simulink model "plant_setup"  (R2022b)
settings: Solver=VariableStepAuto  StartTime=0.0  StopTime=10  RelTol=1e-3
model workspace (MAT data in the model file):
  T_max = Simulink.Parameter
  T_max.Value = 10
  T_max.Description = 'maximum allowable torque command'
  T_max.DataType = 'auto'
  T_max.DocUnits = 'N*m'
  T_max.Complexity = 'real'
  T_max.Dimensions = [1 1]
  bw = Simulink.Parameter
  bw.Value = 0.24
  bw.Description = 'Distance between the two drive wheels'
  bw.DataType = 'auto'
  bw.DocUnits = 'm'
  bw.Complexity = 'real'
  bw.Dimensions = [1 1]
  k_D = Simulink.Parameter
  k_D.Value = 1
  k_D.DataType = 'auto'
  k_D.Complexity = 'real'
  k_D.Dimensions = [1 1]
  k_P = Simulink.Parameter
  k_P.Value = Simulink.data.Expression
  k_P.Value.ExpressionString = "20*k_D"
  k_P.DataType = 'auto'
  k_P.Complexity = 'real'
  k_P.Dimensions = -1
  r_turn = Simulink.Parameter
  r_turn.Value = 0.2
  r_turn.Description = 'Minimum turn radius of the car'
  r_turn.DataType = 'auto'
  r_turn.Min = 0
  r_turn.DocUnits = 'm'
  r_turn.Complexity = 'real'
  r_turn.Dimensions = [1 1]
  r_wheel = Simulink.Parameter
  r_wheel.Value = 0.11
  r_wheel.Description = 'Wheel radius'
  r_wheel.DataType = 'auto'
  r_wheel.DocUnits = 'm'
  r_wheel.Complexity = 'real'
  r_wheel.Dimensions = [1 1]
  v_base = Simulink.Parameter
  v_base.Value = 0.5
  v_base.Description = 'base wheel speed (m/s) used for turns
    | v_base = w_turn_max 8 bw/2'
  v_base.DataType = 'auto'
  v_base.DocUnits = 'm/s'
  v_base.Complexity = 'real'
  v_base.Dimensions = [1 1]
  v_max = Simulink.Parameter
  v_max.Value = 1
  v_max.Description = 'max car speed in m/s'
  v_max.DataType = 'auto'
  v_max.DocUnits = 'm/s'
  v_max.Complexity = 'real'
  v_max.Dimensions = [1 1]
  w_max = Simulink.Parameter
  w_max.Value = Simulink.data.Expression
  w_max.Value.ExpressionString = "9.0909*v_max"
  w_max.Description = 'max wheel speed in rad/s
    | w_max = v_max/r_wheel'
  w_max.DataType = 'auto'
  w_max.DocUnits = 'rad/s'
  w_max.Complexity = 'real'
  w_max.Dimensions = -1
  w_turn_max = Simulink.Parameter
  w_turn_max.Value = 4
  w_turn_max.Description = 'max turning speed of car in rad/s
    | w_turn_max = w_max * r_wheel/bw'
  w_turn_max.DataType = 'auto'
  w_turn_max.DocUnits = 'rad/s'
  w_turn_max.Complexity = 'real'
  w_turn_max.Dimensions = [1 1]
undefined symbols (not defined in the file or in its folder): duration, effort, index, joint_name, left_wheel_hinge, model_name, pioneer2dx, right_wheel_hinge
libraries: robotgazebolib x21, robotcorelib x1, simulink x1
settings Model: Creator=22546723@sun.ac.za  LastModifiedBy=22546723@sun.ac.za

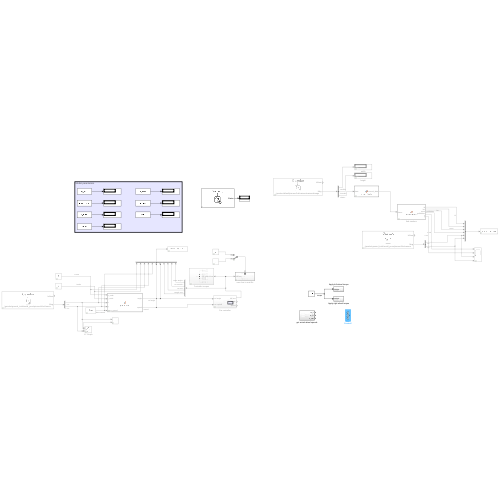
[thumbnail: Simulink's stored preview of the top-level diagram]
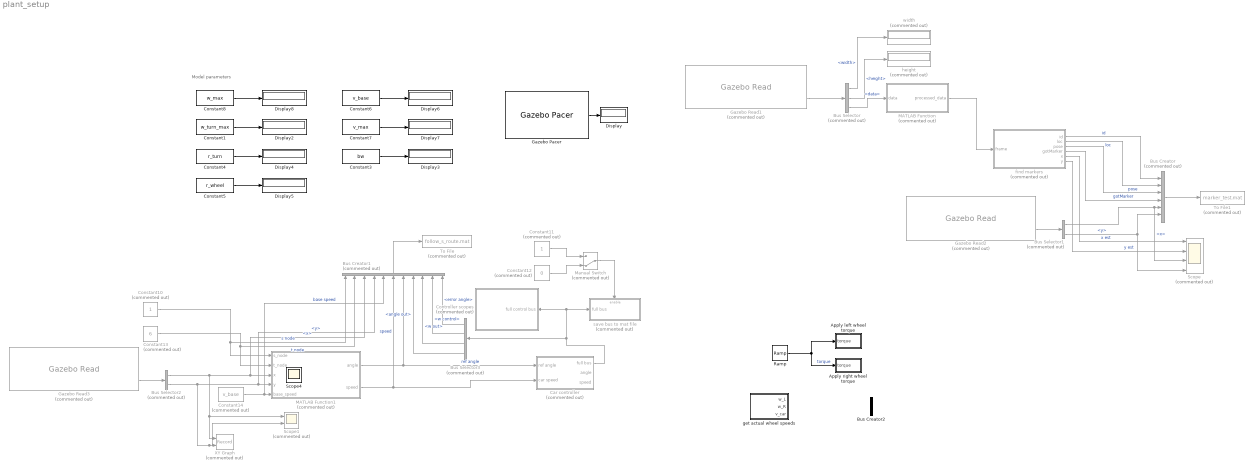
== system plant_setup ==
  note: Model parameters
  Apply left wheel torque : Subsystem
  Apply right wheel torque : Subsystem
  Bus Creator : BusCreator  Commented=on  Inputs=6
  Bus Creator1 : BusCreator  Commented=on  Inputs=11
  Bus Creator2 : BusCreator  Inputs=2
  Bus Selector : BusSelector  Commented=on  OutputSignals=width,height,data
  Bus Selector1 : BusSelector  Commented=on  OutputSignals=position.x,position.y
  Bus Selector2 : BusSelector  Commented=on  OutputSignals=position.x,position.y
  Bus Selector3 : BusSelector  Commented=on  OutputSignals=error angle,w control,w out,angle out
  Car controller : Subsystem  Commented=on
  Constant1 : Constant  Value=w_turn_max
  Constant10 : Constant  Commented=on
  Constant11 : Constant  Commented=on
  Constant12 : Constant  Commented=on  Value=0
  Constant13 : Constant  Commented=on  Value=6
  Constant14 : Constant  Commented=on  Value=v_base
  Constant3 : Constant  Value=bw
  Constant4 : Constant  Value=r_turn
  Constant5 : Constant  Value=r_wheel
  Constant6 : Constant  Value=v_base
  Constant7 : Constant  Value=v_max
  Constant8 : Constant  Value=w_max
  Controller scopes : Subsystem  Commented=on
      settings: PortSchema="{\"entries\":[{\"content\":{\"sides\":[{\"content\":{\"connectorIds\":[]},\"type\":\"ConnectorPlacement.EquallySpacedRectSide\",\"uuid\":\"333996ec-a739-4064-b7cd-e5a785ad06b0\"},{\"content\":{\"connectorIds\":[\"In1\"],\"side\":\"RIGHT\"},\"type\":\"ConnectorPlacement.EquallySpacedRectSide\",\"uuid\":\"5c2099fd-2913-4b55-a92e-2fa47d7778a9\"},{\"content\":{\"connectorIds\":[],\"side\":\"TOP\"},\"type\":\"ConnectorPlacement.EquallySpacedRectSide\",\"uuid\":\"27960070-26ba-4880-ac4a-dbd824c43cf7\"}]},\"type\":\"ConnectorPlacement.EquallySpacedConnector\",\"uuid\":\"80cd80e5-3dd6-4d73-8038-72b1cdb99f2f\"}],\"packageUris\":[\"http://schema.mathworks.com/mf0/Connector/R2020b\"],\"version\":\"1.0\"}"
  Display{,2..8} (8 alike) : Display
  Gazebo Pacer : robotgazebolib/Gazebo Pacer  ResetBehavior=Reset Gazebo simulation time  SampleTime=0.001
  Gazebo Read1 : robotgazebolib/Gazebo Read  Commented=on  topicSource=From Gazebo  topic=/gazebo/default/pioneer2dx/camera/camera/image  messageType=gazebo_msgs/Image  sampleTime=0.001  fixedAxisBusStatus=off  jointAxisCount=2
  Gazebo Read2 : robotgazebolib/Gazebo Read  Commented=on  topicSource=From Gazebo  topic=/gazebo/ground_truth/world_pose/pioneer2dx/camera  messageType=gazebo_msgs/Pose  sampleTime=0.001  fixedAxisBusStatus=off  jointAxisCount=2
  Gazebo Read3 : robotgazebolib/Gazebo Read  Commented=on  topicSource=From Gazebo  topic=/gazebo/ground_truth/world_pose/pioneer2dx/chassis  messageType=gazebo_msgs/Pose  sampleTime=0.001  fixedAxisBusStatus=off  jointAxisCount=2
  MATLAB Function : MATLAB Function  Commented=on  TreatAsAtomicUnit=on
  MATLAB Function1 : MATLAB Function  Commented=on  TreatAsAtomicUnit=on
  Manual Switch : ManualSwitch  Commented=on  CurrentSetting=0
  Ramp : simulink/Sources/Ramp  slope=1  start=0  InitialOutput=0
  Scope : Scope  Commented=on  NumInputPorts=4
  Scope1 : Scope  Commented=on  NumInputPorts=2
  To File : ToFile  Commented=on  Filename=follow_s_route.mat  MatrixName=data  SaveFormat=Timeseries
  To File1 : ToFile  Commented=on  Filename=marker_test.mat  MatrixName=data  SaveFormat=Timeseries
  XY Graph : Record  Commented=on  FileSettingsInternal="{\"entries\":[{\"content\":{\"excelSettings\":{\"content\":{},\"type\":\"Streamout.ExcelSettings\"}},\"type\":\"Streamout.FileSettingStorage\",\"uuid\":\"0a0b0592-9645-4dd3-85ce-6b555624b077\"}],\"packageUris\":[\"http://schema.mathworks.com/mf0/streamout_blocks/R2020a\"],\"version\":\"1.0\"}"  Layout=[1 1]  SignalsInternal="{\"entries\":[{\"content\":{\"signals\":[{\"content\":{\"blockPath\":[\"plant_setup/XY Graph\"],\"channel\":[],\"dimensions\":[1],\"domain\":\"plant_setup/XY Graph\",\"lineColor\":\"#a2142f\",\"plots\":[1],\"port\":1,\"sid\":[],\"signalID\":8,\"signalName\":\"<x>\"},\"type\":\"RecordBlkView.Signal\",\"uuid\":\"999196a1-9528-4da5-9067-52614dff8acd\"},{\"content\":{\"blockPath\":[\"plant_setup/XY Graph\"],\"channel\":[],\"dimensions\":[1],\"domain\":\"plant_setup/XY Graph\",\"lineColor\":\"#139fff\",\"plots\":[1],\"port\":2,\"sid\":[],\"signalID\":11,\"signalName\":\"<y>\"},\"type\":\"RecordBlkView.Signal\",\"uuid\":\"a6f77fcf-062b-42f5-9d76-fad9be37ea72\"}]},\"type\":\"RecordBlkView.InputSignals\",\"uuid\":\"03c2072b-3f6b-465e-b664-df38b8c2c7b2\"}],\"packageUris\":[\"http://schema.mathworks.com/mf0/streamout_blocks/R2020a\"],\"version\":\"1.0\"}"  VisualizationBindings="{\"xyplotplugin\":{\"info\":[{\"series\":[{\"bindingParametersList\":[{\"parameter\":\"X-Axis\",\"signalID\":8,\"signalName\":\"<x>\"},{\"parameter\":\"Y-Axis\",\"signalID\":11,\"signalName\":\"<y>\"}],\"seriesID\":29853}],\"subplotID\":1}]}}"  CompatibilityTag=XY
  find markers : MATLAB Function  Commented=on  TreatAsAtomicUnit=on
  get actual wheel speeds : Subsystem
  height : Display  Commented=on
  save bus to mat file : Subsystem  Commented=on  TreatAsAtomicUnit=on
  width : Display  Commented=on
  Scope4 : Scope
  wires:
  Gazebo Pacer/1 -> Display/1
  Constant1/1 -> Display2/1
  Constant3/1 -> Display3/1
  Constant4/1 -> Display4/1
  Constant5/1 -> Display5/1
  Constant6/1 -> Display6/1
  Constant7/1 -> Display7/1
  Constant8/1 -> Display8/1
  Car controller/1(full bus) -> Bus Selector3/1, save bus to mat file/1(full bus), Controller scopes/1(full control bus)
  Gazebo Read1/2 -> Bus Selector/1
  Bus Selector/3 -> MATLAB Function/1(data)  "<data>"
  Gazebo Read2/2 -> Bus Selector1/1
  find markers/3(pose) -> Bus Creator/3  "pose"
  find markers/4(gotMarker) -> Bus Creator/4  "gotMarker"
  Bus Selector1/1 -> Scope/3, Bus Creator/5  "<x>"
  Bus Selector1/2 -> Scope/4, Bus Creator/6  "<y>"
  MATLAB Function/1(processed_data) -> find markers/1(frame)
  Bus Creator/1 -> To File1/1
  find markers/2(loc) -> Bus Creator/2  "loc"
  find markers/1(id) -> Bus Creator/1  "id"
  Constant11/1 -> Manual Switch/1
  Constant12/1 -> Manual Switch/2
  Manual Switch/1 -> save bus to mat file/Enable
  Bus Selector/1 -> width/1  "<width>"
  Bus Selector/2 -> height/1  "<height>"
  find markers/5(x) -> Scope/1  "x est"
  find markers/6(y) -> Scope/2  "y est"
  Constant10/1 -> MATLAB Function1/1(s_node), Bus Creator1/1  "s node"
  Constant13/1 -> MATLAB Function1/2(t_node), Bus Creator1/2  "t node"
  MATLAB Function1/2(speed) -> Bus Creator1/6, Car controller/2(car speed)  "speed"
  Constant14/1 -> Bus Creator1/5, MATLAB Function1/5(base_speed)  "base speed"
  Gazebo Read3/2 -> Bus Selector2/1
  Bus Selector2/1 -> Scope1/1, XY Graph/1, MATLAB Function1/3(x), Bus Creator1/3  "<x>"
  Bus Selector2/2 -> Scope1/2, XY Graph/2, MATLAB Function1/4(y), Bus Creator1/4  "<y>"
  MATLAB Function1/1(angle) -> Bus Creator1/7, Car controller/1(ref angle)  "ref angle"
  Bus Selector3/1 -> Bus Creator1/11  "<error angle>"
  Bus Selector3/2 -> Bus Creator1/10  "<w control>"
  Bus Selector3/3 -> Bus Creator1/9  "<w out>"
  Bus Selector3/4 -> Bus Creator1/8  "<angle out>"
  Bus Creator1/1 -> To File/1
  Ramp/1 -> Apply right wheel torque/1(torque), Apply left wheel torque/1(torque)  "torque"

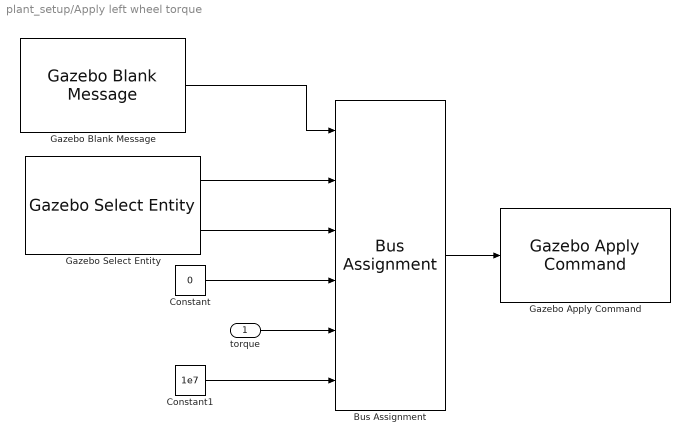
== system plant_setup/Apply left wheel torque ==
  torque : Inport  SampleTime=0.001
  Bus Assignment : BusAssignment  AssignedSignals=model_name,joint_name,index,effort,duration.nano_seconds
  Constant : Constant  Value=0  OutDataTypeStr=uint32  SampleTime=0.001
  Constant1 : Constant  Value=1e7  SampleTime=0.001
  Gazebo Apply Command : robotgazebolib/Gazebo Apply Command  cmdType=ApplyJointTorque  sampleTime=0.001
  Gazebo Blank Message : robotgazebolib/Gazebo Blank Message  msgType=ApplyJointTorque  sampleTime=0.001  busName='Gazebo_SL_Bus_gazebo_msgs_ApplyJointTorque'
  Gazebo Select Entity : robotgazebolib/Gazebo Select Entity  modelElemName=pioneer2dx/left_wheel_hinge  outputArraySize=128  OutputLabel=Joint  SelectType=Joint
  wires:
  Gazebo Select Entity/1 -> Bus Assignment/2
  Bus Assignment/1 -> Gazebo Apply Command/1
  Gazebo Blank Message/1 -> Bus Assignment/1
  Constant/1 -> Bus Assignment/4
  Gazebo Select Entity/2 -> Bus Assignment/3
  Constant1/1 -> Bus Assignment/6
  torque/1 -> Bus Assignment/5

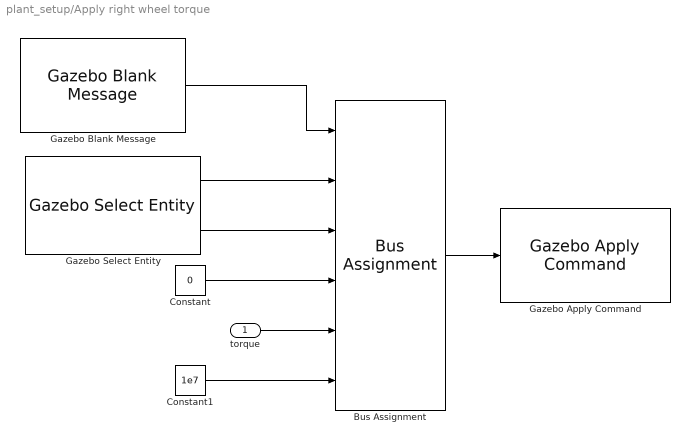
== system plant_setup/Apply right wheel torque ==
  torque : Inport  SampleTime=0.001
  Bus Assignment : BusAssignment  AssignedSignals=model_name,joint_name,index,effort,duration.nano_seconds
  Constant : Constant  Value=0  OutDataTypeStr=uint32  SampleTime=0.001
  Constant1 : Constant  Value=1e7  SampleTime=0.001
  Gazebo Apply Command : robotgazebolib/Gazebo Apply Command  cmdType=ApplyJointTorque  sampleTime=0.001
  Gazebo Blank Message : robotgazebolib/Gazebo Blank Message  msgType=ApplyJointTorque  sampleTime=0.001  busName='Gazebo_SL_Bus_gazebo_msgs_ApplyJointTorque'
  Gazebo Select Entity : robotgazebolib/Gazebo Select Entity  modelElemName=pioneer2dx/right_wheel_hinge  outputArraySize=128  OutputLabel=Joint  SelectType=Joint
  wires:
  Gazebo Select Entity/1 -> Bus Assignment/2
  Bus Assignment/1 -> Gazebo Apply Command/1
  Gazebo Blank Message/1 -> Bus Assignment/1
  Constant/1 -> Bus Assignment/4
  Gazebo Select Entity/2 -> Bus Assignment/3
  Constant1/1 -> Bus Assignment/6
  torque/1 -> Bus Assignment/5

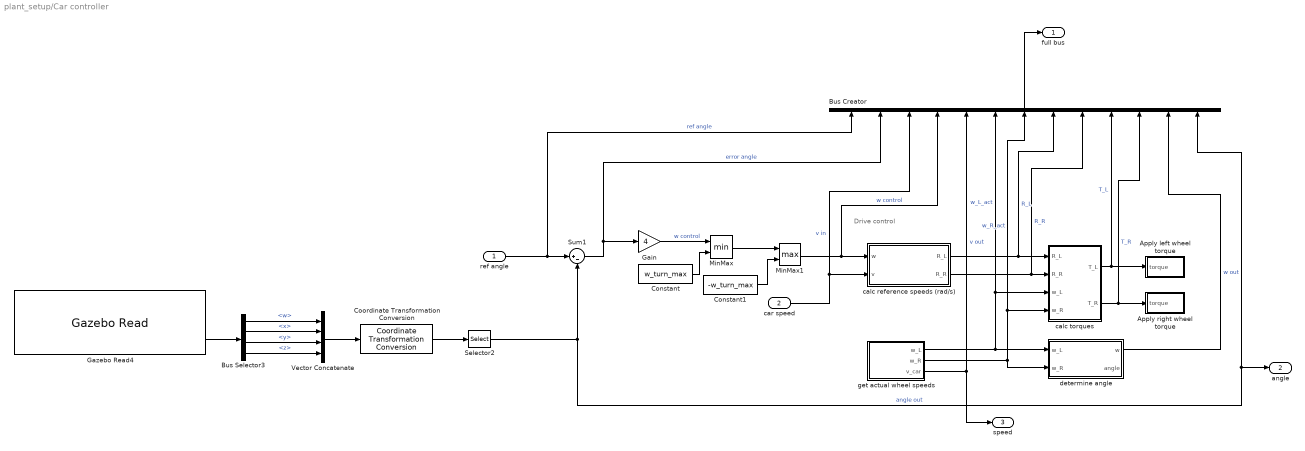
== system plant_setup/Car controller ==
  note: Drive control
  ref angle : Inport
  car speed : Inport  Port=2
  Apply left wheel torque : Subsystem
  Apply right wheel torque : Subsystem
  Bus Creator : BusCreator  Inputs=13
  Bus Selector3 : BusSelector  OutputSignals=orientation.w,orientation.x,orientation.y,orientation.z
  Constant : Constant  Value=w_turn_max
  Constant1 : Constant  Value=-w_turn_max
  Coordinate Transformation Conversion : robotcorelib/Coordinate Transformation Conversion  InputRepresentation=Quaternion  InputEulerSequence=ZYX  ShowTrVecInputPort=on  OutputRepresentation=Euler Angles  OutputEulerSequence=ZYX  ShowTrVecOutputPort=on  SimulateUsing=Interpreted execution
  Gain : Gain  Gain=4
  Gazebo Read4 : robotgazebolib/Gazebo Read  topicSource=From Gazebo  topic=/gazebo/ground_truth/world_pose/pioneer2dx/chassis  messageType=gazebo_msgs/Pose  sampleTime=0.001  fixedAxisBusStatus=off  jointAxisCount=2
  MinMax : MinMax  Inputs=2
  MinMax1 : MinMax  Function=max  Inputs=2
  Selector2 : Selector  InputPortWidth=3  IndexOptions=Index vector (dialog)  Indices=1  OutputSizes=1
  Sum1 : Sum  Inputs=|+-
  Vector Concatenate : Concatenate  NumInputs=4
  calc reference speeds (rad/s) : Subsystem
  calc torques : Subsystem
  determine angle : Subsystem
  get actual wheel speeds : Subsystem
  full bus : Outport
  angle : Outport  Port=2
  speed : Outport  Port=3
  wires:
  car speed/1 -> calc reference speeds (rad/s)/2(v), Bus Creator/3  "v in"
  Bus Creator/1 -> full bus/1
  calc torques/1(T_L) -> Bus Creator/10, Apply left wheel torque/1(torque)  "T_L"
  get actual wheel speeds/2(w_R) -> determine angle/2(w_R), calc torques/4(w_R), Bus Creator/7  "w_R_act"
  MinMax1/1 -> Bus Creator/4, calc reference speeds (rad/s)/1(w)  "w control"
  calc torques/2(T_R) -> Apply right wheel torque/1(torque), Bus Creator/11  "T_R"
  ref angle/1 -> Sum1/1, Bus Creator/1  "ref angle"
  calc reference speeds (rad/s)/2(R_R) -> calc torques/2(R_R), Bus Creator/9  "R_R"
  determine angle/1(w) -> Bus Creator/12  "w out"
  calc reference speeds (rad/s)/1(R_L) -> calc torques/1(R_L), Bus Creator/8  "R_L"
  get actual wheel speeds/1(w_L) -> determine angle/1(w_L), calc torques/3(w_L), Bus Creator/6  "w_L_act"
  get actual wheel speeds/3(v_car) -> speed/1, Bus Creator/5  "v out"
  Vector Concatenate/1 -> Coordinate Transformation Conversion/1
  Bus Selector3/2 -> Vector Concatenate/2  "<x>"
  Bus Selector3/1 -> Vector Concatenate/1  "<w>"
  Bus Selector3/3 -> Vector Concatenate/3  "<y>"
  Bus Selector3/4 -> Vector Concatenate/4  "<z>"
  Coordinate Transformation Conversion/1 -> Selector2/1
  Gazebo Read4/2 -> Bus Selector3/1
  Selector2/1 -> Sum1/2, Bus Creator/13, angle/1  "angle out"
  Sum1/1 -> Gain/1, Bus Creator/2  "error angle"
  Constant/1 -> MinMax/2
  MinMax/1 -> MinMax1/1
  Constant1/1 -> MinMax1/2
  Gain/1 -> MinMax/1  "w control"

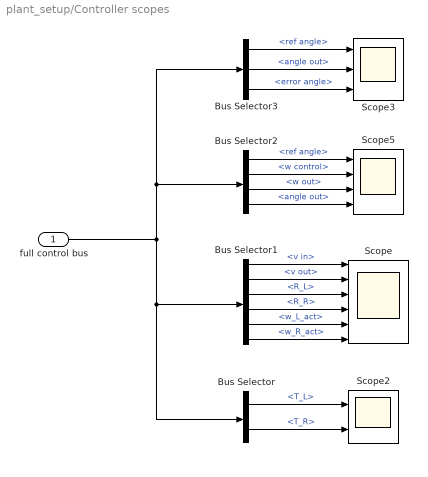
== system plant_setup/Controller scopes ==
  full control bus : Inport
  Bus Selector : BusSelector  OutputSignals=T_L,T_R
  Bus Selector1 : BusSelector  OutputSignals=v in,v out,R_L,R_R,w_L_act,w_R_act
  Bus Selector2 : BusSelector  OutputSignals=ref angle,w control,w out,angle out
  Bus Selector3 : BusSelector  OutputSignals=ref angle,angle out,error angle
  Scope : Scope  NumInputPorts=6
  Scope2 : Scope  NumInputPorts=2
  Scope3 : Scope  NumInputPorts=3
  Scope5 : Scope  NumInputPorts=4
  wires:
  Bus Selector3/2 -> Scope3/2  "<angle out>"
  Bus Selector1/2 -> Scope/2  "<v out>"
  Bus Selector2/1 -> Scope5/1  "<ref angle>"
  Bus Selector3/1 -> Scope3/1  "<ref angle>"
  Bus Selector/2 -> Scope2/2  "<T_R>"
  Bus Selector1/3 -> Scope/3  "<R_L>"
  Bus Selector2/3 -> Scope5/3  "<w out>"
  full control bus/1 -> Bus Selector/1, Bus Selector1/1, Bus Selector2/1, Bus Selector3/1
  Bus Selector1/4 -> Scope/4  "<R_R>"
  Bus Selector2/2 -> Scope5/2  "<w control>"
  Bus Selector/1 -> Scope2/1  "<T_L>"
  Bus Selector2/4 -> Scope5/4  "<angle out>"
  Bus Selector3/3 -> Scope3/3  "<error angle>"
  Bus Selector1/5 -> Scope/5  "<w_L_act>"
  Bus Selector1/1 -> Scope/1  "<v in>"
  Bus Selector1/6 -> Scope/6  "<w_R_act>"

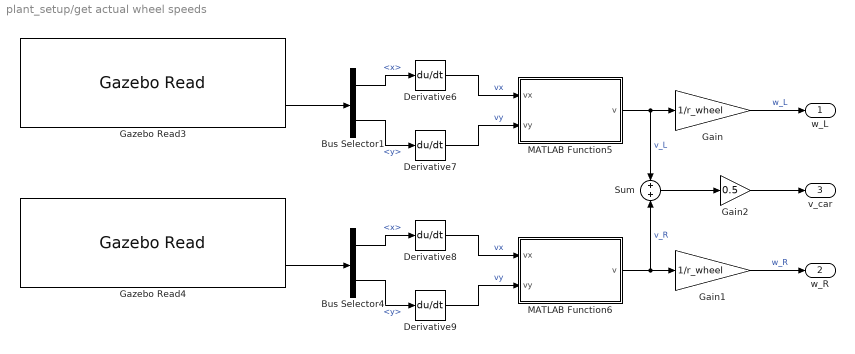
== system plant_setup/get actual wheel speeds ==
  Bus Selector1 : BusSelector  OutputSignals=position.x,position.y
  Bus Selector4 : BusSelector  OutputSignals=position.x,position.y
  Derivative{6..9} (4 alike) : Derivative
  Gain : Gain  Gain=1/r_wheel
  Gain1 : Gain  Gain=1/r_wheel
  Gain2 : Gain  Gain=0.5
  Gazebo Read3 : robotgazebolib/Gazebo Read  topicSource=From Gazebo  topic=/gazebo/ground_truth/world_pose/pioneer2dx/left_wheel  messageType=gazebo_msgs/Pose  sampleTime=0.001  fixedAxisBusStatus=off  jointAxisCount=2
  Gazebo Read4 : robotgazebolib/Gazebo Read  topicSource=From Gazebo  topic=/gazebo/ground_truth/world_pose/pioneer2dx/right_wheel  messageType=gazebo_msgs/Pose  sampleTime=0.001  fixedAxisBusStatus=off  jointAxisCount=2
  MATLAB Function5 : MATLAB Function  TreatAsAtomicUnit=on
  MATLAB Function6 : MATLAB Function  TreatAsAtomicUnit=on
  Sum : Sum  Inputs=+|+
  w_L : Outport
  w_R : Outport  Port=2
  v_car : Outport  Port=3
  wires:
  Bus Selector4/1 -> Derivative8/1  "<x>"
  Bus Selector4/2 -> Derivative9/1  "<y>"
  Derivative8/1 -> MATLAB Function6/1(vx)  "vx"
  Derivative9/1 -> MATLAB Function6/2(vy)  "vy"
  Derivative6/1 -> MATLAB Function5/1(vx)  "vx"
  Gazebo Read3/2 -> Bus Selector1/1
  Bus Selector1/1 -> Derivative6/1  "<x>"
  Bus Selector1/2 -> Derivative7/1  "<y>"
  Gazebo Read4/2 -> Bus Selector4/1
  Derivative7/1 -> MATLAB Function5/2(vy)  "vy"
  MATLAB Function5/1(v) -> Sum/1, Gain/1  "v_L"
  Gain/1 -> w_L/1  "w_L"
  MATLAB Function6/1(v) -> Sum/2, Gain1/1  "v_R"
  Gain1/1 -> w_R/1  "w_R"
  Sum/1 -> Gain2/1
  Gain2/1 -> v_car/1

== system plant_setup/save bus to mat file ==
  full bus : Inport
  Enable : EnablePort
  Bus Selector : BusSelector  OutputSignals=angle out
  To File : ToFile  Commented=on  Filename=Results/full_control/blank.mat  MatrixName=data  SaveFormat=Timeseries
  To Workspace : ToWorkspace  VariableName=angle_out  SaveFormat=Timeseries  SampleTime=-1
  wires:
  full bus/1 -> Bus Selector/1, To File/1
  Bus Selector/1 -> To Workspace/1  "<angle out>"

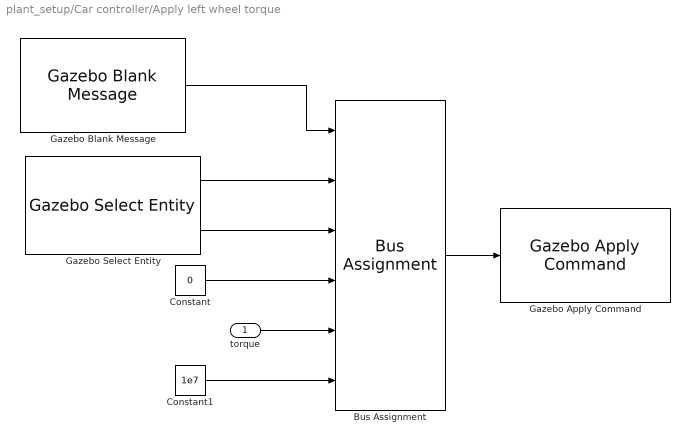
== system plant_setup/Car controller/Apply left wheel torque ==
  torque : Inport  SampleTime=0.001
  Bus Assignment : BusAssignment  AssignedSignals=model_name,joint_name,index,effort,duration.nano_seconds
  Constant : Constant  Value=0  OutDataTypeStr=uint32  SampleTime=0.001
  Constant1 : Constant  Value=1e7  SampleTime=0.001
  Gazebo Apply Command : robotgazebolib/Gazebo Apply Command  cmdType=ApplyJointTorque  sampleTime=0.001
  Gazebo Blank Message : robotgazebolib/Gazebo Blank Message  msgType=ApplyJointTorque  sampleTime=0.001  busName='Gazebo_SL_Bus_gazebo_msgs_ApplyJointTorque'
  Gazebo Select Entity : robotgazebolib/Gazebo Select Entity  modelElemName=pioneer2dx/left_wheel_hinge  outputArraySize=128  OutputLabel=Joint  SelectType=Joint
  wires:
  Gazebo Select Entity/1 -> Bus Assignment/2
  Bus Assignment/1 -> Gazebo Apply Command/1
  Gazebo Blank Message/1 -> Bus Assignment/1
  Constant/1 -> Bus Assignment/4
  Gazebo Select Entity/2 -> Bus Assignment/3
  Constant1/1 -> Bus Assignment/6
  torque/1 -> Bus Assignment/5

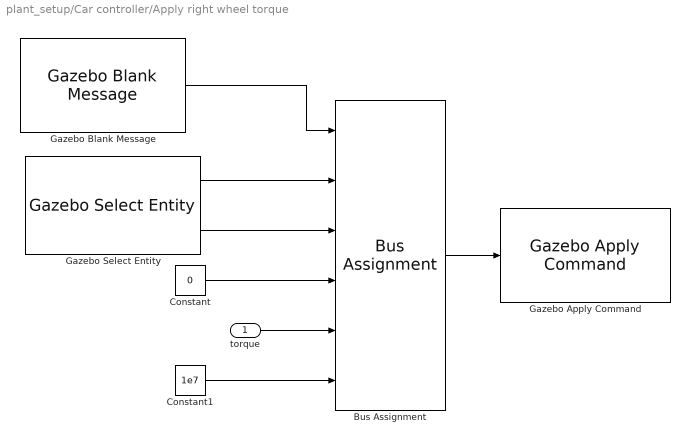
== system plant_setup/Car controller/Apply right wheel torque ==
  torque : Inport  SampleTime=0.001
  Bus Assignment : BusAssignment  AssignedSignals=model_name,joint_name,index,effort,duration.nano_seconds
  Constant : Constant  Value=0  OutDataTypeStr=uint32  SampleTime=0.001
  Constant1 : Constant  Value=1e7  SampleTime=0.001
  Gazebo Apply Command : robotgazebolib/Gazebo Apply Command  cmdType=ApplyJointTorque  sampleTime=0.001
  Gazebo Blank Message : robotgazebolib/Gazebo Blank Message  msgType=ApplyJointTorque  sampleTime=0.001  busName='Gazebo_SL_Bus_gazebo_msgs_ApplyJointTorque'
  Gazebo Select Entity : robotgazebolib/Gazebo Select Entity  modelElemName=pioneer2dx/right_wheel_hinge  outputArraySize=128  OutputLabel=Joint  SelectType=Joint
  wires:
  Gazebo Select Entity/1 -> Bus Assignment/2
  Bus Assignment/1 -> Gazebo Apply Command/1
  Gazebo Blank Message/1 -> Bus Assignment/1
  Constant/1 -> Bus Assignment/4
  Gazebo Select Entity/2 -> Bus Assignment/3
  Constant1/1 -> Bus Assignment/6
  torque/1 -> Bus Assignment/5

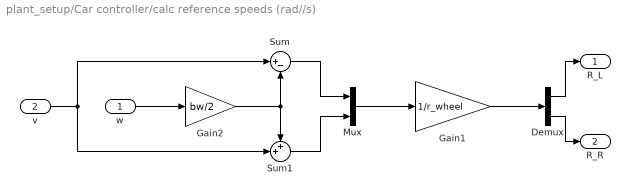
== system plant_setup/Car controller/calc reference speeds (rad//s) ==
  w : Inport
  v : Inport  Port=2
  Demux : Demux  Outputs=2
  Gain1 : Gain  Gain=1/r_wheel
  Gain2 : Gain  Gain=bw/2
  Mux : Mux  Inputs=2
  Sum : Sum  Inputs=|+-
  Sum1 : Sum  Inputs=++|
  R_L : Outport
  R_R : Outport  Port=2
  wires:
  v/1 -> Sum/1, Sum1/2
  Sum/1 -> Mux/1
  Demux/1 -> R_L/1
  Gain2/1 -> Sum1/1, Sum/2
  Sum1/1 -> Mux/2
  Gain1/1 -> Demux/1
  Mux/1 -> Gain1/1
  w/1 -> Gain2/1
  Demux/2 -> R_R/1

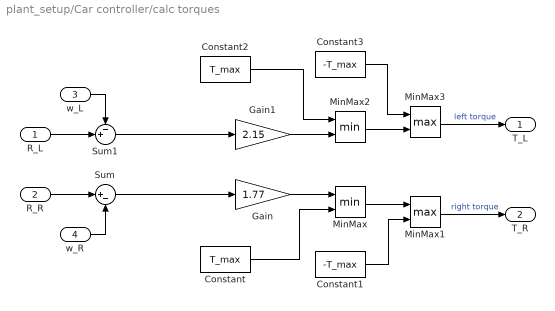
== system plant_setup/Car controller/calc torques ==
  R_L : Inport
  R_R : Inport  Port=2
  w_L : Inport  Port=3
  w_R : Inport  Port=4
  Constant : Constant  Value=T_max
  Constant1 : Constant  Value=-T_max
  Constant2 : Constant  Value=T_max
  Constant3 : Constant  Value=-T_max
  Gain : Gain  Gain=1.77
  Gain1 : Gain  Gain=2.15
  MinMax : MinMax  Inputs=2
  MinMax1 : MinMax  Function=max  Inputs=2
  MinMax2 : MinMax  Inputs=2
  MinMax3 : MinMax  Function=max  Inputs=2
  Sum : Sum  Inputs=|+-
  Sum1 : Sum  Inputs=-+|
  T_L : Outport
  T_R : Outport  Port=2
  wires:
  Sum/1 -> Gain/1
  w_R/1 -> Sum/2
  Sum1/1 -> Gain1/1
  R_R/1 -> Sum/1
  w_L/1 -> Sum1/1
  R_L/1 -> Sum1/2
  Gain/1 -> MinMax/1
  Constant/1 -> MinMax/2
  MinMax/1 -> MinMax1/1
  Constant1/1 -> MinMax1/2
  Gain1/1 -> MinMax2/2
  Constant2/1 -> MinMax2/1
  MinMax2/1 -> MinMax3/2
  Constant3/1 -> MinMax3/1
  MinMax3/1 -> T_L/1  "left torque"
  MinMax1/1 -> T_R/1  "right torque"

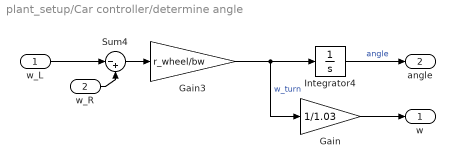
== system plant_setup/Car controller/determine angle ==
  w_L : Inport
  w_R : Inport  Port=2
  Gain : Gain  Gain=1/1.03
  Gain3 : Gain  Gain=r_wheel/bw
  Integrator4 : Integrator
  Sum4 : Sum  Inputs=|-+
  w : Outport
  angle : Outport  Port=2
  wires:
  Gain3/1 -> Gain/1, Integrator4/1  "w_turn"
  Sum4/1 -> Gain3/1
  w_R/1 -> Sum4/2
  Integrator4/1 -> angle/1  "angle"
  w_L/1 -> Sum4/1
  Gain/1 -> w/1

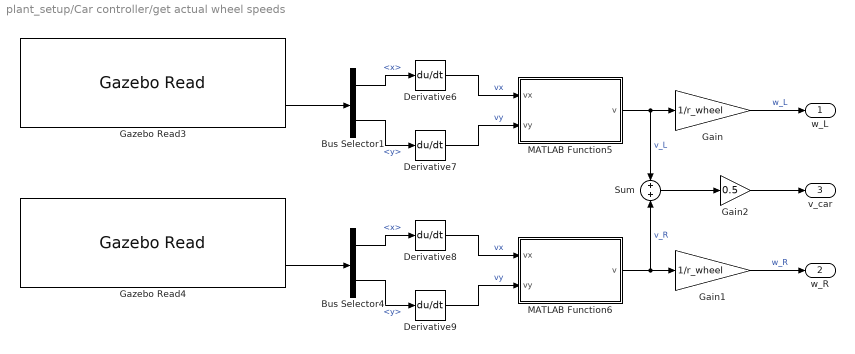
== system plant_setup/Car controller/get actual wheel speeds ==
  Bus Selector1 : BusSelector  OutputSignals=position.x,position.y
  Bus Selector4 : BusSelector  OutputSignals=position.x,position.y
  Derivative{6..9} (4 alike) : Derivative
  Gain : Gain  Gain=1/r_wheel
  Gain1 : Gain  Gain=1/r_wheel
  Gain2 : Gain  Gain=0.5
  Gazebo Read3 : robotgazebolib/Gazebo Read  topicSource=From Gazebo  topic=/gazebo/ground_truth/world_pose/pioneer2dx/left_wheel  messageType=gazebo_msgs/Pose  sampleTime=0.001  fixedAxisBusStatus=off  jointAxisCount=2
  Gazebo Read4 : robotgazebolib/Gazebo Read  topicSource=From Gazebo  topic=/gazebo/ground_truth/world_pose/pioneer2dx/right_wheel  messageType=gazebo_msgs/Pose  sampleTime=0.001  fixedAxisBusStatus=off  jointAxisCount=2
  MATLAB Function5 : MATLAB Function  TreatAsAtomicUnit=on
  MATLAB Function6 : MATLAB Function  TreatAsAtomicUnit=on
  Sum : Sum  Inputs=+|+
  w_L : Outport
  w_R : Outport  Port=2
  v_car : Outport  Port=3
  wires:
  Bus Selector4/1 -> Derivative8/1  "<x>"
  Bus Selector4/2 -> Derivative9/1  "<y>"
  Derivative8/1 -> MATLAB Function6/1(vx)  "vx"
  Derivative9/1 -> MATLAB Function6/2(vy)  "vy"
  Derivative6/1 -> MATLAB Function5/1(vx)  "vx"
  Gazebo Read3/2 -> Bus Selector1/1
  Bus Selector1/1 -> Derivative6/1  "<x>"
  Bus Selector1/2 -> Derivative7/1  "<y>"
  Gazebo Read4/2 -> Bus Selector4/1
  Derivative7/1 -> MATLAB Function5/2(vy)  "vy"
  MATLAB Function5/1(v) -> Sum/1, Gain/1  "v_L"
  Gain/1 -> w_L/1  "w_L"
  MATLAB Function6/1(v) -> Sum/2, Gain1/1  "v_R"
  Gain1/1 -> w_R/1  "w_R"
  Sum/1 -> Gain2/1
  Gain2/1 -> v_car/1

== matlab function plant_setup/find markers ==
  data: frame input; id output; loc output; pose output; gotMarker output; x output; y output
function [id, loc, pose, gotMarker, x, y] = findMarkers(frame) % [status, id, loc, pose, gotMarker] = findMarkers(frame, params)
% persistent intrinsics
% coder.extrinsic('readAprilTag')
% 
% status = 0;     % 0 : params empty | 1 : params not empty
% tag_family = "tag36h11";
% tag_size = 0.1; %10cm
% 
% id = 0;
% loc = 0;
% pose = 0;
% gotMarker = 0;
% 
% disp(size(frame))
% 
% if isempty(intrinsics)&&(~isempty(params))
% 
%     focal_length = params(1:2);
%     principal_point = params(3:4);
%     image_size = [2464, 3280]; %params(5:6);
%     radial_distortion = params(7:8);
% 
%     intrinsics = cameraIntrinsics(focal_length, ...
%         principal_point, image_size, 'RadialDistortion', ...
%         radial_distortion);
% 
% end
% 
% if ~isempty(intrinsics)
%     frame = undistortImage(frame, intrinsics, OutputView='same');
%     [id, loc, pose] = readAprilTag(frame, tag_family, intrinsics, tag_size);
% 
%     if isempty(loc)
%         gotMarker = 0;
%     else
%         gotMarker = 1;
%     end
% end
% 
% if ~isempty(params)
%     status = 1;
% end


persistent cam_helper
coder.extrinsic("camHelper")
coder.extrinsic("getMarkers")

max_markers = 1;
id = 404; % zeros(max_markers, 1, 1);
loc = zeros(4, 2, 1);
pose = zeros(4, 4, 1);
%pose = rigidtform3d(A);
x = 0;
y = 0;

gotMarker = 0;

if isempty(cam_helper)
    cam_helper = camHelper;
end

[id, loc, pose, gotMarker, x, y] = getMarkers(cam_helper, frame);

== matlab function plant_setup/MATLAB Function ==
  data: data input; processed_data output
function processed_data=processVideo(data)
% the camera sends a 1200*600*3 data signal. Simulink receives it as a 1-D
% array

width = 3280;
height = 2464;
z = 3;

processed_data = zeros(height, width, z, 'uint8');

if ~isempty(data) && ~isscalar(data)

    indexBase = (1:z:width*height*z)';
    index = zeros(numel(indexBase), z);

    for i=1:z
        index(:, i) = indexBase + i - 1;
    end

    temp = reshape(data(index), width, height, z);
    processed_data = permute(temp, [2 1 3]);

end

== matlab function plant_setup/MATLAB Function1 ==
  data: angle output; s_node input; t_node input; x input; y input; base_speed input; speed output
function [angle, speed] = getRoute(s_node, t_node, x, y, base_speed)
persistent routePlanner
persistent segment_num
persistent reached_target
coder.extrinsic("route_planner")
coder.extrinsic("get_ref_array")

brake_point = 0.5; %distance from t_node where braking should start
node_radius = 0.1; 

if isempty(reached_target)
    reached_target = 0;
end

xt = 0;
yt = 0;
len = 0;
angle = 0;
speed = 0;

%speed = base_speed;

%

if isempty(routePlanner)
    routePlanner = route_planner();
end

if isempty(segment_num)
    segment_num = 1;
end

ref_signal = get_ref_array(routePlanner, s_node, t_node);
len = size(ref_signal,2);

xt = ref_signal(3, segment_num);
yt = ref_signal(4, segment_num);

if reached_target==0
    speed = base_speed;
    angle = atan((yt-y)/(xt-x));
end

dist_to_next = sqrt((yt-y)^2 + (xt-x)^2);

if (segment_num==len)&&(dist_to_next<=brake_point)&&(reached_target==0)
    speed = base_speed*dist_to_next/brake_point;
end



if dist_to_next < node_radius
    if (segment_num==len)
        %segment_num = 1;
        reached_target = 1;
    else
        segment_num = segment_num+1;
    end
end

== matlab function plant_setup/Car controller/get actual wheel speeds/MATLAB Function5 ==
  settings: updateMethod=DISCRETE
  data: vx input; v output; vy input
function v = detSpeed(vx, vy)
persistent prev_x
persistent prev_y

if isempty(prev_x)
    prev_x = 0;
end

if isempty(prev_y)
    prev_y = 0;
end

if abs(prev_x - vx)>1
    vx = prev_x;
else
    prev_x = vx;
end

if abs(prev_y - vy)>1
    vy = prev_y;
else 
    prev_y = vy;
end

v = sqrt(vx^2 + vy^2);

== matlab function plant_setup/get actual wheel speeds/MATLAB Function5 ==
  settings: updateMethod=DISCRETE
  data: vx input; v output; vy input
function v = detSpeed(vx, vy)
persistent prev_x
persistent prev_y

if isempty(prev_x)
    prev_x = 0;
end

if isempty(prev_y)
    prev_y = 0;
end

if abs(prev_x - vx)>1
    vx = prev_x;
else
    prev_x = vx;
end

if abs(prev_y - vy)>1
    vy = prev_y;
else 
    prev_y = vy;
end

v = sqrt(vx^2 + vy^2);

== matlab function plant_setup/get actual wheel speeds/MATLAB Function6 ==
  settings: updateMethod=DISCRETE
  data: vx input; v output; vy input
function v = detSpeed(vx, vy)
persistent prev_x
persistent prev_y

if isempty(prev_x)
    prev_x = 0;
end

if isempty(prev_y)
    prev_y = 0;
end

if abs(prev_x - vx)>1
    vx = prev_x;
else
    prev_x = vx;
end

if abs(prev_y - vy)>1
    vy = prev_y;
else 
    prev_y = vy;
end

v = sqrt(vx^2 + vy^2);

== matlab function plant_setup/Car controller/get actual wheel speeds/MATLAB Function6 ==
  settings: updateMethod=DISCRETE
  data: vx input; v output; vy input
function v = detSpeed(vx, vy)
persistent prev_x
persistent prev_y

if isempty(prev_x)
    prev_x = 0;
end

if isempty(prev_y)
    prev_y = 0;
end

if abs(prev_x - vx)>1
    vx = prev_x;
else
    prev_x = vx;
end

if abs(prev_y - vy)>1
    vy = prev_y;
else 
    prev_y = vy;
end

v = sqrt(vx^2 + vy^2);
